simulink model "APCS"  (R2023a)
settings: Solver=VariableStepAuto  StartTime=0.0  StopTime=10.0  RelTol=1e-3
settings Model: Creator=asd19005  LastModifiedBy=aan18022

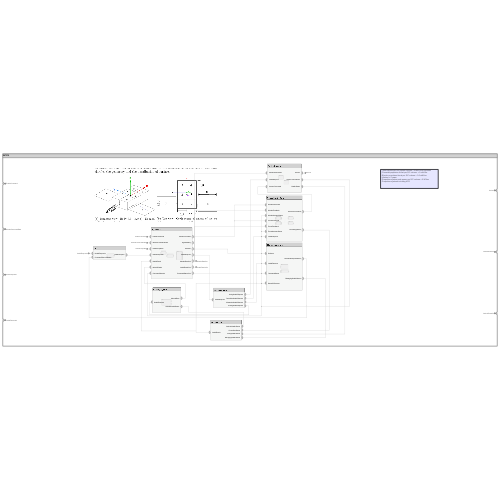
[thumbnail: Simulink's stored preview of the top-level diagram]
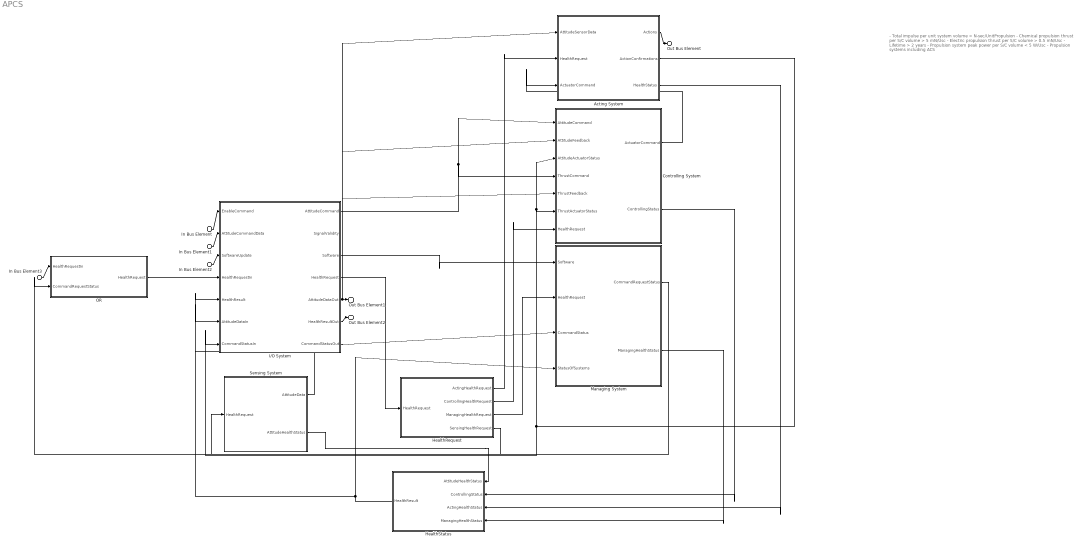
== system APCS ==
  note: - Total impulse per unit system volume > N-sec/UnitPropulsion
      | - Chemical propulsion thrust per S/C volume  > 5 mN/Usc
      | - Electric propulsion thrust per S/C volume > 0.5 mN/Usc
      | - Lifetime > 2 years
      | - Propulsion system peak power per S/C volume < 5 W/Usc
      | - Propulsion systems including ACS
  In Bus Element : Inport  PortName=EnableCommand
  In Bus Element1 : Inport  Port=2  PortName=AttitudeCommandData
  In Bus Element2 : Inport  Port=3  PortName=SoftwareUpdate
  In Bus Element3 : Inport  Port=4  PortName=HealthRequestIn
  Acting System : Subsystem
      settings: PortSchema="{\"entries\":[{\"content\":{\"headerSize\":26,\"margin\":15,\"minimumSpacing\":25,\"sides\":[{\"content\":{\"connectorIds\":[\"In1\",\"In2\",\"In3\"]},\"type\":\"ConnectorPlacement.EquallySpacedRectSide\",\"uuid\":\"fe9a0813-768f-43cf-a7a7-a35f6718a35e\"},{\"content\":{\"connectorIds\":[\"Out1\",\"Out2\",\"Out3\"],\"side\":\"RIGHT\"},\"type\":\"ConnectorPlacement.EquallySpacedRectSide\",\"uuid\":\"83a5fda2-f793-4516-8295-8e256804f86f\"},{\"content\":{\"side\":\"TOP\"},\"type\":\"ConnectorPlacement.EquallySpacedRectSide\",\"uuid\":\"9f7bc7bd-a98b-401f-acf1-cfd6a0f445f8\"}]},\"type\":\"ConnectorPlacement.EquallySpacedConnector\",\"uuid\":\"2641b729-a1f9-4d54-83a2-7f405081950a\"}],\"packageUris\":[\"http://schema.mathworks.com/mf0/Connector/R2020b\"],\"version\":\"1.0\"}"
  Controlling System : Subsystem
      settings: PortSchema="{\"entries\":[{\"content\":{\"headerSize\":26,\"margin\":15,\"minimumSpacing\":25,\"sides\":[{\"content\":{\"connectorIds\":[\"In1\",\"In5\",\"In3\",\"In2\",\"In6\",\"In4\",\"In7\"]},\"type\":\"ConnectorPlacement.EquallySpacedRectSide\",\"uuid\":\"fe9a0813-768f-43cf-a7a7-a35f6718a35e\"},{\"content\":{\"connectorIds\":[\"Out1\",\"Out2\"],\"side\":\"RIGHT\"},\"type\":\"ConnectorPlacement.EquallySpacedRectSide\",\"uuid\":\"83a5fda2-f793-4516-8295-8e256804f86f\"},{\"content\":{\"side\":\"TOP\"},\"type\":\"ConnectorPlacement.EquallySpacedRectSide\",\"uuid\":\"9f7bc7bd-a98b-401f-acf1-cfd6a0f445f8\"}]},\"type\":\"ConnectorPlacement.EquallySpacedConnector\",\"uuid\":\"2641b729-a1f9-4d54-83a2-7f405081950a\"}],\"packageUris\":[\"http://schema.mathworks.com/mf0/Connector/R2020b\"],\"version\":\"1.0\"}"
  HealthRequest : Subsystem
      settings: PortSchema="{\"entries\":[{\"content\":{\"headerSize\":26,\"margin\":15,\"minimumSpacing\":25,\"sides\":[{\"content\":{\"connectorIds\":[\"In1\"]},\"type\":\"ConnectorPlacement.EquallySpacedRectSide\",\"uuid\":\"fe9a0813-768f-43cf-a7a7-a35f6718a35e\"},{\"content\":{\"connectorIds\":[\"Out4\",\"Out1\",\"Out2\",\"Out3\"],\"side\":\"RIGHT\"},\"type\":\"ConnectorPlacement.EquallySpacedRectSide\",\"uuid\":\"83a5fda2-f793-4516-8295-8e256804f86f\"},{\"content\":{\"side\":\"TOP\"},\"type\":\"ConnectorPlacement.EquallySpacedRectSide\",\"uuid\":\"9f7bc7bd-a98b-401f-acf1-cfd6a0f445f8\"}]},\"type\":\"ConnectorPlacement.EquallySpacedConnector\",\"uuid\":\"2641b729-a1f9-4d54-83a2-7f405081950a\"}],\"packageUris\":[\"http://schema.mathworks.com/mf0/Connector/R2020b\"],\"version\":\"1.0\"}"
  HealthStatus : Subsystem
      settings: PortSchema="{\"entries\":[{\"content\":{\"headerSize\":26,\"margin\":15,\"minimumSpacing\":25,\"sides\":[{\"content\":{\"connectorIds\":[\"Out1\"]},\"type\":\"ConnectorPlacement.EquallySpacedRectSide\",\"uuid\":\"fe9a0813-768f-43cf-a7a7-a35f6718a35e\"},{\"content\":{\"connectorIds\":[\"In1\",\"In2\",\"In3\",\"In4\"],\"side\":\"RIGHT\"},\"type\":\"ConnectorPlacement.EquallySpacedRectSide\",\"uuid\":\"83a5fda2-f793-4516-8295-8e256804f86f\"},{\"content\":{\"side\":\"TOP\"},\"type\":\"ConnectorPlacement.EquallySpacedRectSide\",\"uuid\":\"9f7bc7bd-a98b-401f-acf1-cfd6a0f445f8\"}]},\"type\":\"ConnectorPlacement.EquallySpacedConnector\",\"uuid\":\"2641b729-a1f9-4d54-83a2-7f405081950a\"}],\"packageUris\":[\"http://schema.mathworks.com/mf0/Connector/R2020b\"],\"version\":\"1.0\"}"
  I/O System : Subsystem
      settings: PortSchema="{\"entries\":[{\"content\":{\"headerSize\":26,\"margin\":15,\"minimumSpacing\":25,\"sides\":[{\"content\":{\"connectorIds\":[\"In1\",\"In2\",\"In3\",\"In4\",\"In5\",\"In6\",\"In7\"]},\"type\":\"ConnectorPlacement.EquallySpacedRectSide\",\"uuid\":\"fe9a0813-768f-43cf-a7a7-a35f6718a35e\"},{\"content\":{\"connectorIds\":[\"Out1\",\"Out2\",\"Out3\",\"Out4\",\"Out5\",\"Out6\",\"Out7\"],\"side\":\"RIGHT\"},\"type\":\"ConnectorPlacement.EquallySpacedRectSide\",\"uuid\":\"83a5fda2-f793-4516-8295-8e256804f86f\"},{\"content\":{\"side\":\"TOP\"},\"type\":\"ConnectorPlacement.EquallySpacedRectSide\",\"uuid\":\"9f7bc7bd-a98b-401f-acf1-cfd6a0f445f8\"}]},\"type\":\"ConnectorPlacement.EquallySpacedConnector\",\"uuid\":\"2641b729-a1f9-4d54-83a2-7f405081950a\"}],\"packageUris\":[\"http://schema.mathworks.com/mf0/Connector/R2020b\"],\"version\":\"1.0\"}"
  Managing System : Subsystem
      settings: PortSchema="{\"entries\":[{\"content\":{\"headerSize\":26,\"margin\":15,\"minimumSpacing\":25,\"sides\":[{\"content\":{\"connectorIds\":[\"In1\",\"In2\",\"In3\",\"In4\"]},\"type\":\"ConnectorPlacement.EquallySpacedRectSide\",\"uuid\":\"fe9a0813-768f-43cf-a7a7-a35f6718a35e\"},{\"content\":{\"connectorIds\":[\"Out1\",\"Out2\"],\"side\":\"RIGHT\"},\"type\":\"ConnectorPlacement.EquallySpacedRectSide\",\"uuid\":\"83a5fda2-f793-4516-8295-8e256804f86f\"},{\"content\":{\"side\":\"TOP\"},\"type\":\"ConnectorPlacement.EquallySpacedRectSide\",\"uuid\":\"9f7bc7bd-a98b-401f-acf1-cfd6a0f445f8\"}]},\"type\":\"ConnectorPlacement.EquallySpacedConnector\",\"uuid\":\"2641b729-a1f9-4d54-83a2-7f405081950a\"}],\"packageUris\":[\"http://schema.mathworks.com/mf0/Connector/R2020b\"],\"version\":\"1.0\"}"
  OR : Subsystem
      settings: PortSchema="{\"entries\":[{\"content\":{\"headerSize\":26,\"margin\":15,\"minimumSpacing\":25,\"sides\":[{\"content\":{\"connectorIds\":[\"In2\",\"In1\"]},\"type\":\"ConnectorPlacement.EquallySpacedRectSide\",\"uuid\":\"fe9a0813-768f-43cf-a7a7-a35f6718a35e\"},{\"content\":{\"connectorIds\":[\"Out1\"],\"side\":\"RIGHT\"},\"type\":\"ConnectorPlacement.EquallySpacedRectSide\",\"uuid\":\"83a5fda2-f793-4516-8295-8e256804f86f\"},{\"content\":{\"side\":\"TOP\"},\"type\":\"ConnectorPlacement.EquallySpacedRectSide\",\"uuid\":\"9f7bc7bd-a98b-401f-acf1-cfd6a0f445f8\"}]},\"type\":\"ConnectorPlacement.EquallySpacedConnector\",\"uuid\":\"2641b729-a1f9-4d54-83a2-7f405081950a\"}],\"packageUris\":[\"http://schema.mathworks.com/mf0/Connector/R2020b\"],\"version\":\"1.0\"}"
  Sensing System : Subsystem
      settings: PortSchema="{\"entries\":[{\"content\":{\"headerSize\":26,\"margin\":15,\"minimumSpacing\":25,\"sides\":[{\"content\":{\"connectorIds\":[\"In1\"]},\"type\":\"ConnectorPlacement.EquallySpacedRectSide\",\"uuid\":\"fe9a0813-768f-43cf-a7a7-a35f6718a35e\"},{\"content\":{\"connectorIds\":[\"Out1\",\"Out2\"],\"side\":\"RIGHT\"},\"type\":\"ConnectorPlacement.EquallySpacedRectSide\",\"uuid\":\"83a5fda2-f793-4516-8295-8e256804f86f\"},{\"content\":{\"side\":\"TOP\"},\"type\":\"ConnectorPlacement.EquallySpacedRectSide\",\"uuid\":\"9f7bc7bd-a98b-401f-acf1-cfd6a0f445f8\"}]},\"type\":\"ConnectorPlacement.EquallySpacedConnector\",\"uuid\":\"2641b729-a1f9-4d54-83a2-7f405081950a\"}],\"packageUris\":[\"http://schema.mathworks.com/mf0/Connector/R2020b\"],\"version\":\"1.0\"}"
  Out Bus Element : Outport  PortName=Actions
  Out Bus Element2 : Outport  Port=2  PortName=HealthResultOut
  Out Bus Element1 : Outport  Port=3  PortName=AttitudeDataOut
  wires:
  In Bus Element/1 -> I/O System/1(EnableCommand)
  In Bus Element1/1 -> I/O System/2(AttitudeCommandData)
  In Bus Element2/1 -> I/O System/3(SoftwareUpdate)
  I/O System/1(AttitudeCommand) -> Controlling System/1(AttitudeCommand), Controlling System/2(ThrustCommand)
  I/O System/3(Software) -> Managing System/1(Software)
  Sensing System/1(AttitudeData) -> I/O System/6(AttitudeDataIn)
  Acting System/2(ActionConfirmations) -> Controlling System/3(AttitudeActuatorStatus), Controlling System/4(ThrustActuatorStatus), I/O System/7(CommandStatusIn)
  I/O System/5(AttitudeDataOut) -> Controlling System/5(AttitudeFeedback), Acting System/1(AttitudeSensorData), Controlling System/6(ThrustFeedback), Out Bus Element1/1
  I/O System/7(CommandStatusOut) -> Managing System/3(CommandStatus)
  Controlling System/1(ActuatorCommand) -> Acting System/3(ActuatorCommand)
  Acting System/1(Actions) -> Out Bus Element/1
  I/O System/6(HealthResultOut) -> Out Bus Element2/1
  I/O System/4(HealthRequest) -> HealthRequest/1(HealthRequest)
  HealthRequest/1(ControllingHealthRequest) -> Controlling System/7(HealthRequest)
  HealthRequest/2(ManagingHealthRequest) -> Managing System/2(HealthRequest)
  HealthRequest/4(ActingHealthRequest) -> Acting System/2(HealthRequest)
  HealthStatus/1(HealthResult) -> Managing System/4(StatusOfSystems), I/O System/5(HealthResult)
  HealthRequest/3(SensingHealthRequest) -> Sensing System/1(HealthRequest)
  Acting System/3(HealthStatus) -> HealthStatus/3(ActingHealthStatus)
  Managing System/2(ManagingHealthStatus) -> HealthStatus/4(ManagingHealthStatus)
  Controlling System/2(ControllingStatus) -> HealthStatus/2(ControllingStatus)
  In Bus Element3/1 -> OR/2(HealthRequestIn)
  Managing System/1(CommandRequestStatus) -> OR/1(CommandRequestStatus)
  OR/1(HealthRequest) -> I/O System/4(HealthRequestIn)
  Sensing System/2(AttitudeHealthStatus) -> HealthStatus/1(AttitudeHealthStatus)

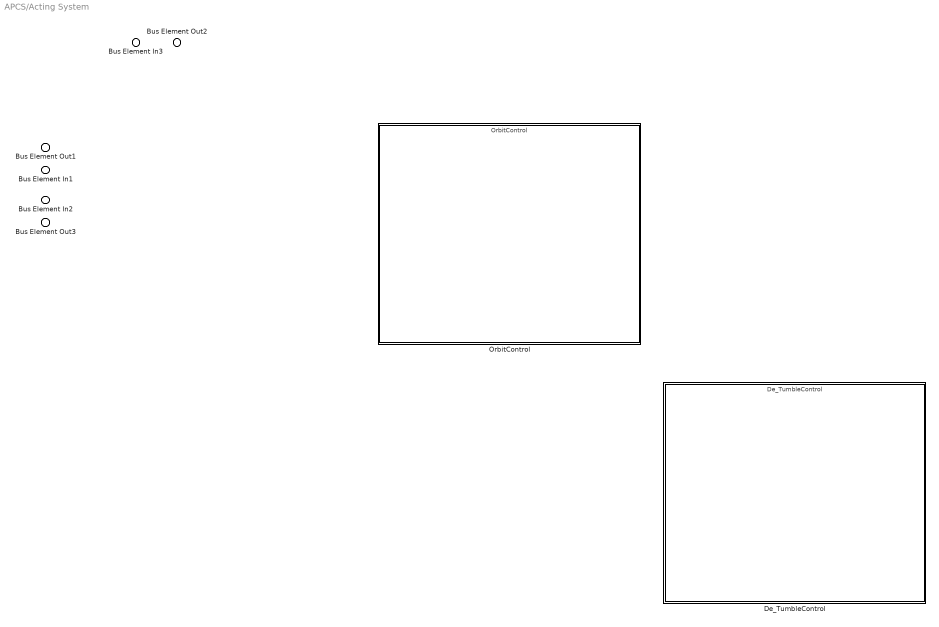
== system APCS/Acting System ==
  Bus Element In1 : Inport  PortName=AttitudeSensorData
  Bus Element In3 : Inport  Port=2  PortName=HealthRequest
  Bus Element In2 : Inport  Port=3  PortName=ActuatorCommand
  De_TumbleControl : ModelReference  ModelNameDialog=De_TumbleControl  SimulationMode=Normal  ModelReferenceVersion=1.0
      settings: PortSchema="{\"entries\":[{\"content\":{\"headerSize\":38,\"margin\":15,\"minimumSpacing\":25,\"sides\":[{\"content\":{},\"type\":\"ConnectorPlacement.EquallySpacedRectSide\",\"uuid\":\"e3457a29-b43c-4933-8a11-68e017a647c4\"},{\"content\":{\"side\":\"RIGHT\"},\"type\":\"ConnectorPlacement.EquallySpacedRectSide\",\"uuid\":\"7dfa2731-a543-4e50-aed6-e868771da571\"},{\"content\":{\"side\":\"TOP\"},\"type\":\"ConnectorPlacement.EquallySpacedRectSide\",\"uuid\":\"66e179e8-d7ed-4bc5-a0bd-f79bc464d9fe\"}]},\"type\":\"ConnectorPlacement.EquallySpacedConnector\",\"uuid\":\"61bb093a-de12-4127-8c6a-9ae2c62bada7\"}],\"packageUris\":[\"http://schema.mathworks.com/mf0/Connector/R2020b\"],\"version\":\"1.0\"}"
  OrbitControl : ModelReference  ModelNameDialog=OrbitControl  SimulationMode=Normal  ModelReferenceVersion=1.0
      settings: PortSchema="{\"entries\":[{\"content\":{\"headerSize\":38,\"margin\":15,\"minimumSpacing\":25,\"sides\":[{\"content\":{},\"type\":\"ConnectorPlacement.EquallySpacedRectSide\",\"uuid\":\"e3457a29-b43c-4933-8a11-68e017a647c4\"},{\"content\":{\"side\":\"RIGHT\"},\"type\":\"ConnectorPlacement.EquallySpacedRectSide\",\"uuid\":\"7dfa2731-a543-4e50-aed6-e868771da571\"},{\"content\":{\"side\":\"TOP\"},\"type\":\"ConnectorPlacement.EquallySpacedRectSide\",\"uuid\":\"66e179e8-d7ed-4bc5-a0bd-f79bc464d9fe\"}]},\"type\":\"ConnectorPlacement.EquallySpacedConnector\",\"uuid\":\"61bb093a-de12-4127-8c6a-9ae2c62bada7\"}],\"packageUris\":[\"http://schema.mathworks.com/mf0/Connector/R2020b\"],\"version\":\"1.0\"}"
  Bus Element Out2 : Outport  PortName=Actions
  Bus Element Out1 : Outport  Port=2  PortName=ActionConfirmations
  Bus Element Out3 : Outport  Port=3  PortName=HealthStatus

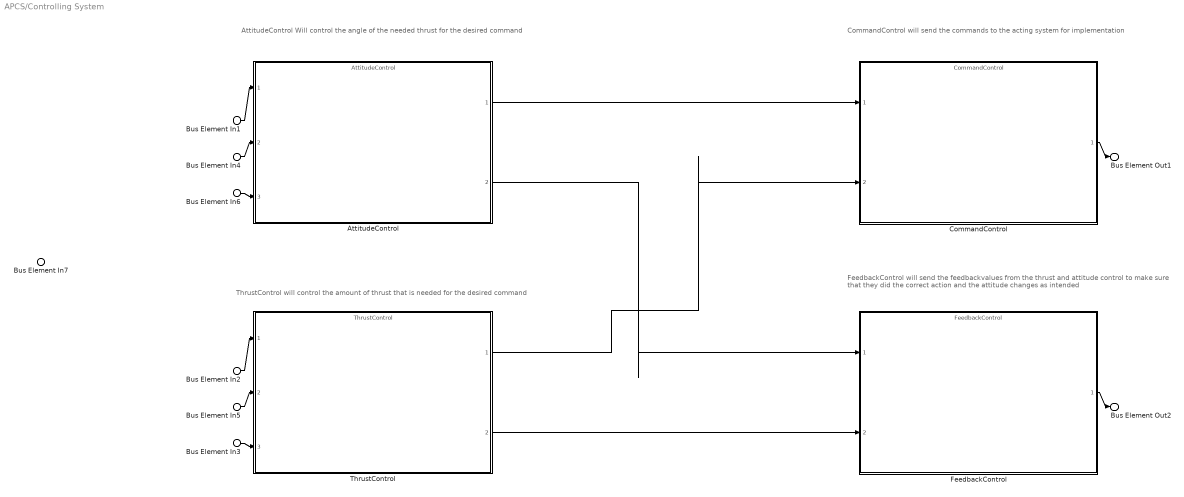
== system APCS/Controlling System ==
  note: CommandControl will send the commands to the acting system for implementation
  note: ThrustControl will control the amount of thrust that is needed for the desired command
  note: AttitudeControl Will control the angle of the needed thrust for the desired command
  note: FeedbackControl will send the feedbackvalues from the thrust and attitude control to make sure that they did the correct action and the attitude changes as intended
  Bus Element In1 : Inport  PortName=AttitudeCommand
  Bus Element In2 : Inport  Port=2  PortName=ThrustCommand
  Bus Element In6 : Inport  Port=3  PortName=AttitudeActuatorStatus
  Bus Element In3 : Inport  Port=4  PortName=ThrustActuatorStatus
  Bus Element In4 : Inport  Port=5  PortName=AttitudeFeedback
  Bus Element In5 : Inport  Port=6  PortName=ThrustFeedback
  Bus Element In7 : Inport  Port=7  PortName=HealthRequest
  AttitudeControl : ModelReference  ModelNameDialog=AttitudeControl.slx  SimulationMode=Normal  ModelReferenceVersion=1.1
      settings: PortSchema="{\"entries\":[{\"content\":{\"headerSize\":38,\"margin\":15,\"minimumSpacing\":25,\"sides\":[{\"content\":{\"connectorIds\":[\"In1\",\"In2\",\"In3\"]},\"type\":\"ConnectorPlacement.EquallySpacedRectSide\",\"uuid\":\"e3457a29-b43c-4933-8a11-68e017a647c4\"},{\"content\":{\"connectorIds\":[\"Out1\",\"Out2\"],\"side\":\"RIGHT\"},\"type\":\"ConnectorPlacement.EquallySpacedRectSide\",\"uuid\":\"7dfa2731-a543-4e50-aed6-e868771da571\"},{\"content\":{\"side\":\"TOP\"},\"type\":\"ConnectorPlacement.EquallySpacedRectSide\",\"uuid\":\"66e179e8-d7ed-4bc5-a0bd-f79bc464d9fe\"}]},\"type\":\"ConnectorPlacement.EquallySpacedConnector\",\"uuid\":\"61bb093a-de12-4127-8c6a-9ae2c62bada7\"}],\"packageUris\":[\"http://schema.mathworks.com/mf0/Connector/R2020b\"],\"version\":\"1.0\"}"
  CommandControl : ModelReference  ModelNameDialog=CommandControl  SimulationMode=Normal  ModelReferenceVersion=1.1
      settings: PortSchema="{\"entries\":[{\"content\":{\"headerSize\":38,\"margin\":15,\"minimumSpacing\":25,\"sides\":[{\"content\":{\"connectorIds\":[\"In1\",\"In2\"]},\"type\":\"ConnectorPlacement.EquallySpacedRectSide\",\"uuid\":\"e3457a29-b43c-4933-8a11-68e017a647c4\"},{\"content\":{\"connectorIds\":[\"Out1\"],\"side\":\"RIGHT\"},\"type\":\"ConnectorPlacement.EquallySpacedRectSide\",\"uuid\":\"7dfa2731-a543-4e50-aed6-e868771da571\"},{\"content\":{\"side\":\"TOP\"},\"type\":\"ConnectorPlacement.EquallySpacedRectSide\",\"uuid\":\"66e179e8-d7ed-4bc5-a0bd-f79bc464d9fe\"}]},\"type\":\"ConnectorPlacement.EquallySpacedConnector\",\"uuid\":\"61bb093a-de12-4127-8c6a-9ae2c62bada7\"}],\"packageUris\":[\"http://schema.mathworks.com/mf0/Connector/R2020b\"],\"version\":\"1.0\"}"
  FeedbackControl : ModelReference  ModelNameDialog=FeedbackControl  SimulationMode=Normal  ModelReferenceVersion=1.1
      settings: PortSchema="{\"entries\":[{\"content\":{\"headerSize\":38,\"margin\":15,\"minimumSpacing\":25,\"sides\":[{\"content\":{\"connectorIds\":[\"In1\",\"In2\"]},\"type\":\"ConnectorPlacement.EquallySpacedRectSide\",\"uuid\":\"e3457a29-b43c-4933-8a11-68e017a647c4\"},{\"content\":{\"connectorIds\":[\"Out1\"],\"side\":\"RIGHT\"},\"type\":\"ConnectorPlacement.EquallySpacedRectSide\",\"uuid\":\"7dfa2731-a543-4e50-aed6-e868771da571\"},{\"content\":{\"side\":\"TOP\"},\"type\":\"ConnectorPlacement.EquallySpacedRectSide\",\"uuid\":\"66e179e8-d7ed-4bc5-a0bd-f79bc464d9fe\"}]},\"type\":\"ConnectorPlacement.EquallySpacedConnector\",\"uuid\":\"61bb093a-de12-4127-8c6a-9ae2c62bada7\"}],\"packageUris\":[\"http://schema.mathworks.com/mf0/Connector/R2020b\"],\"version\":\"1.0\"}"
  ThrustControl : ModelReference  ModelNameDialog=ThrustControl  SimulationMode=Normal  ModelReferenceVersion=1.1
      settings: PortSchema="{\"entries\":[{\"content\":{\"headerSize\":38,\"margin\":15,\"minimumSpacing\":25,\"sides\":[{\"content\":{\"connectorIds\":[\"In1\",\"In2\",\"In3\"]},\"type\":\"ConnectorPlacement.EquallySpacedRectSide\",\"uuid\":\"e3457a29-b43c-4933-8a11-68e017a647c4\"},{\"content\":{\"connectorIds\":[\"Out1\",\"Out2\"],\"side\":\"RIGHT\"},\"type\":\"ConnectorPlacement.EquallySpacedRectSide\",\"uuid\":\"7dfa2731-a543-4e50-aed6-e868771da571\"},{\"content\":{\"side\":\"TOP\"},\"type\":\"ConnectorPlacement.EquallySpacedRectSide\",\"uuid\":\"66e179e8-d7ed-4bc5-a0bd-f79bc464d9fe\"}]},\"type\":\"ConnectorPlacement.EquallySpacedConnector\",\"uuid\":\"61bb093a-de12-4127-8c6a-9ae2c62bada7\"}],\"packageUris\":[\"http://schema.mathworks.com/mf0/Connector/R2020b\"],\"version\":\"1.0\"}"
  Bus Element Out1 : Outport  PortName=ActuatorCommand
  Bus Element Out2 : Outport  Port=2  PortName=ControllingStatus
  wires:
  Bus Element In6/1 -> AttitudeControl/3
  Bus Element In1/1 -> AttitudeControl/1
  Bus Element In4/1 -> AttitudeControl/2
  Bus Element In3/1 -> ThrustControl/3
  Bus Element In2/1 -> ThrustControl/1
  Bus Element In5/1 -> ThrustControl/2
  AttitudeControl/1 -> CommandControl/1
  ThrustControl/1 -> CommandControl/2
  CommandControl/1 -> Bus Element Out1/1
  AttitudeControl/2 -> FeedbackControl/1
  ThrustControl/2 -> FeedbackControl/2
  FeedbackControl/1 -> Bus Element Out2/1

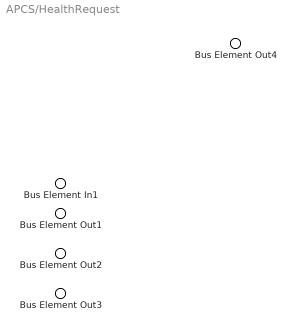
== system APCS/HealthRequest ==
  Bus Element In1 : Inport  PortName=HealthRequest
  Bus Element Out1 : Outport  PortName=ControllingHealthRequest
  Bus Element Out2 : Outport  Port=2  PortName=ManagingHealthRequest
  Bus Element Out4 : Outport  Port=3  PortName=SensingHealthRequest
  Bus Element Out3 : Outport  Port=4  PortName=ActingHealthRequest

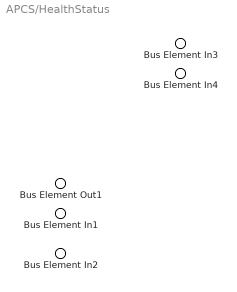
== system APCS/HealthStatus ==
  Bus Element In4 : Inport  PortName=AttitudeHealthStatus
  Bus Element In3 : Inport  Port=2  PortName=ControllingStatus
  Bus Element In1 : Inport  Port=3  PortName=ActingHealthStatus
  Bus Element In2 : Inport  Port=4  PortName=ManagingHealthStatus
  Bus Element Out1 : Outport  PortName=HealthResult

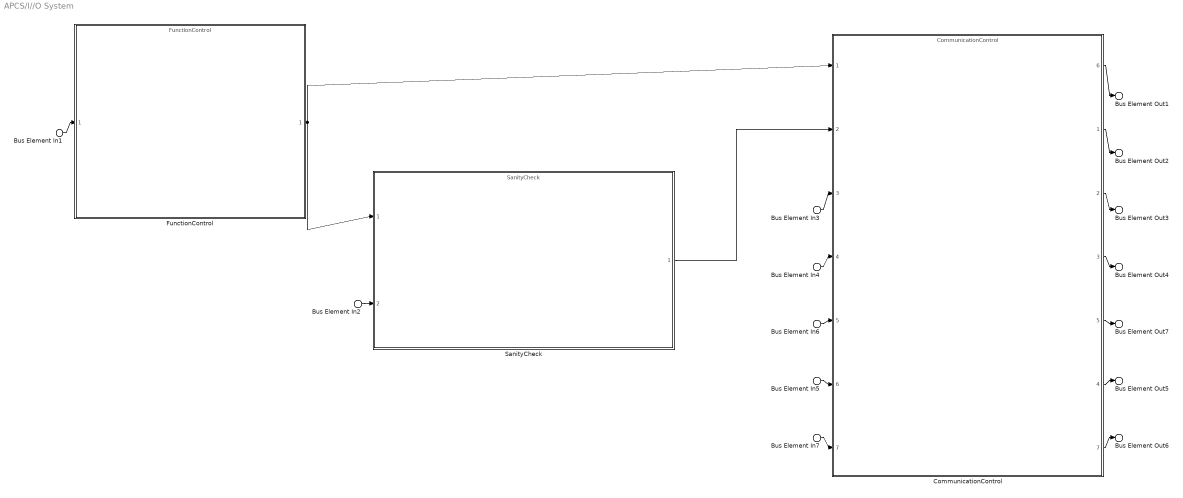
== system APCS/I//O System ==
  Bus Element In1 : Inport  PortName=EnableCommand
  Bus Element In2 : Inport  Port=2  PortName=AttitudeCommandData
  Bus Element In3 : Inport  Port=3  PortName=SoftwareUpdate
  Bus Element In4 : Inport  Port=4  PortName=HealthRequestIn
  Bus Element In6 : Inport  Port=5  PortName=HealthResult
  Bus Element In5 : Inport  Port=6  PortName=AttitudeDataIn
  Bus Element In7 : Inport  Port=7  PortName=CommandStatusIn
  CommunicationControl : ModelReference  ModelNameDialog=CommunicationControl  SimulationMode=Normal  ModelReferenceVersion=1.2
      settings: PortSchema="{\"entries\":[{\"content\":{\"headerSize\":38,\"margin\":15,\"minimumSpacing\":25,\"sides\":[{\"content\":{\"connectorIds\":[\"In1\",\"In2\",\"In3\",\"In4\",\"In5\",\"In6\",\"In7\"]},\"type\":\"ConnectorPlacement.EquallySpacedRectSide\",\"uuid\":\"e3457a29-b43c-4933-8a11-68e017a647c4\"},{\"content\":{\"connectorIds\":[\"Out6\",\"Out1\",\"Out2\",\"Out3\",\"Out5\",\"Out4\",\"Out7\"],\"side\":\"RIGHT\"},\"type\":\"ConnectorPlacement.EquallySpacedRectSide\",\"uuid\":\"7dfa2731-a543-4e50-aed6-e868771da571\"},{\"content\":{\"side\":\"TOP\"},\"type\":\"ConnectorPlacement.EquallySpacedRectSide\",\"uuid\":\"66e179e8-d7ed-4bc5-a0bd-f79bc464d9fe\"}]},\"type\":\"ConnectorPlacement.EquallySpacedConnector\",\"uuid\":\"61bb093a-de12-4127-8c6a-9ae2c62bada7\"}],\"packageUris\":[\"http://schema.mathworks.com/mf0/Connector/R2020b\"],\"version\":\"1.0\"}"
  FunctionControl : ModelReference  ModelNameDialog=FunctionControl  SimulationMode=Normal  ModelReferenceVersion=1.2
      settings: PortSchema="{\"entries\":[{\"content\":{\"headerSize\":38,\"margin\":15,\"minimumSpacing\":25,\"sides\":[{\"content\":{\"connectorIds\":[\"In1\"]},\"type\":\"ConnectorPlacement.EquallySpacedRectSide\",\"uuid\":\"e3457a29-b43c-4933-8a11-68e017a647c4\"},{\"content\":{\"connectorIds\":[\"Out1\"],\"side\":\"RIGHT\"},\"type\":\"ConnectorPlacement.EquallySpacedRectSide\",\"uuid\":\"7dfa2731-a543-4e50-aed6-e868771da571\"},{\"content\":{\"side\":\"TOP\"},\"type\":\"ConnectorPlacement.EquallySpacedRectSide\",\"uuid\":\"66e179e8-d7ed-4bc5-a0bd-f79bc464d9fe\"}]},\"type\":\"ConnectorPlacement.EquallySpacedConnector\",\"uuid\":\"61bb093a-de12-4127-8c6a-9ae2c62bada7\"}],\"packageUris\":[\"http://schema.mathworks.com/mf0/Connector/R2020b\"],\"version\":\"1.0\"}"
  SanityCheck : ModelReference  ModelNameDialog=SanityCheck  SimulationMode=Normal  ModelReferenceVersion=1.2
      settings: PortSchema="{\"entries\":[{\"content\":{\"headerSize\":38,\"margin\":15,\"minimumSpacing\":25,\"sides\":[{\"content\":{\"connectorIds\":[\"In1\",\"In2\"]},\"type\":\"ConnectorPlacement.EquallySpacedRectSide\",\"uuid\":\"e3457a29-b43c-4933-8a11-68e017a647c4\"},{\"content\":{\"connectorIds\":[\"Out1\"],\"side\":\"RIGHT\"},\"type\":\"ConnectorPlacement.EquallySpacedRectSide\",\"uuid\":\"7dfa2731-a543-4e50-aed6-e868771da571\"},{\"content\":{\"side\":\"TOP\"},\"type\":\"ConnectorPlacement.EquallySpacedRectSide\",\"uuid\":\"66e179e8-d7ed-4bc5-a0bd-f79bc464d9fe\"}]},\"type\":\"ConnectorPlacement.EquallySpacedConnector\",\"uuid\":\"61bb093a-de12-4127-8c6a-9ae2c62bada7\"}],\"packageUris\":[\"http://schema.mathworks.com/mf0/Connector/R2020b\"],\"version\":\"1.0\"}"
  Bus Element Out1 : Outport  PortName=AttitudeCommand
  Bus Element Out2 : Outport  Port=2  PortName=SignalValidity
  Bus Element Out3 : Outport  Port=3  PortName=Software
  Bus Element Out4 : Outport  Port=4  PortName=HealthRequest
  Bus Element Out5 : Outport  Port=5  PortName=AttitudeDataOut
  Bus Element Out7 : Outport  Port=6  PortName=HealthResultOut
  Bus Element Out6 : Outport  Port=7  PortName=CommandStatusOut
  wires:
  Bus Element In1/1 -> FunctionControl/1
  FunctionControl/1 -> SanityCheck/1, CommunicationControl/1
  Bus Element In2/1 -> SanityCheck/2
  SanityCheck/1 -> CommunicationControl/2
  Bus Element In5/1 -> CommunicationControl/6
  Bus Element In7/1 -> CommunicationControl/7
  Bus Element In4/1 -> CommunicationControl/4
  Bus Element In6/1 -> CommunicationControl/5
  Bus Element In3/1 -> CommunicationControl/3
  CommunicationControl/6 -> Bus Element Out1/1
  CommunicationControl/4 -> Bus Element Out5/1
  CommunicationControl/7 -> Bus Element Out6/1
  CommunicationControl/3 -> Bus Element Out4/1
  CommunicationControl/5 -> Bus Element Out7/1
  CommunicationControl/1 -> Bus Element Out2/1
  CommunicationControl/2 -> Bus Element Out3/1

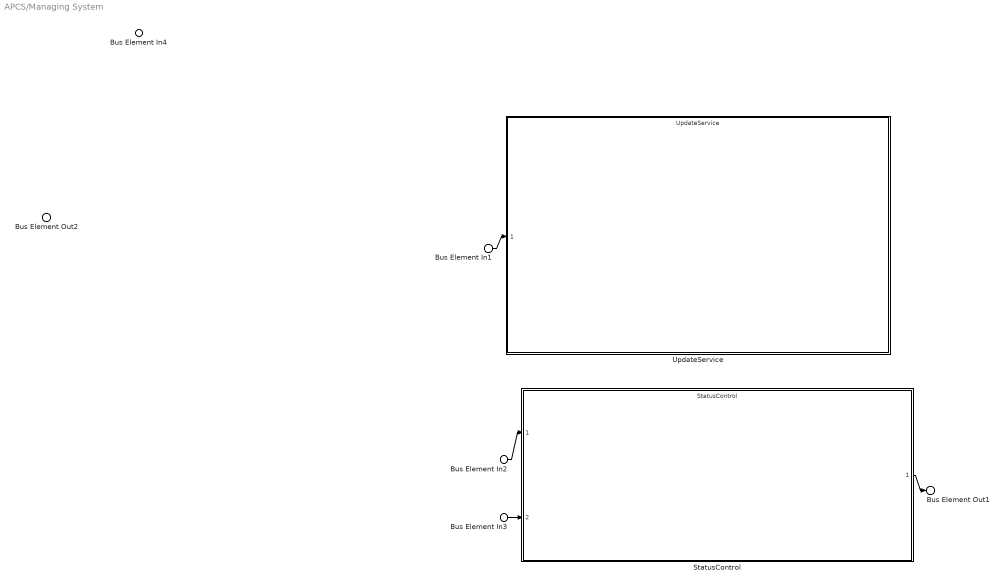
== system APCS/Managing System ==
  Bus Element In1 : Inport  PortName=Software
  Bus Element In4 : Inport  Port=2  PortName=HealthRequest
  Bus Element In2 : Inport  Port=3  PortName=CommandStatus
  Bus Element In3 : Inport  Port=4  PortName=StatusOfSystems
  StatusControl : ModelReference  ModelNameDialog=StatusControl  SimulationMode=Normal  ModelReferenceVersion=1.1
      settings: PortSchema="{\"entries\":[{\"content\":{\"headerSize\":38,\"margin\":15,\"minimumSpacing\":25,\"sides\":[{\"content\":{\"connectorIds\":[\"In1\",\"In2\"]},\"type\":\"ConnectorPlacement.EquallySpacedRectSide\",\"uuid\":\"e3457a29-b43c-4933-8a11-68e017a647c4\"},{\"content\":{\"connectorIds\":[\"Out1\"],\"side\":\"RIGHT\"},\"type\":\"ConnectorPlacement.EquallySpacedRectSide\",\"uuid\":\"7dfa2731-a543-4e50-aed6-e868771da571\"},{\"content\":{\"side\":\"TOP\"},\"type\":\"ConnectorPlacement.EquallySpacedRectSide\",\"uuid\":\"66e179e8-d7ed-4bc5-a0bd-f79bc464d9fe\"}]},\"type\":\"ConnectorPlacement.EquallySpacedConnector\",\"uuid\":\"61bb093a-de12-4127-8c6a-9ae2c62bada7\"}],\"packageUris\":[\"http://schema.mathworks.com/mf0/Connector/R2020b\"],\"version\":\"1.0\"}"
  UpdateService : ModelReference  ModelNameDialog=UpdateService  SimulationMode=Normal  ModelReferenceVersion=1.1
      settings: PortSchema="{\"entries\":[{\"content\":{\"headerSize\":38,\"margin\":15,\"minimumSpacing\":25,\"sides\":[{\"content\":{\"connectorIds\":[\"In1\"]},\"type\":\"ConnectorPlacement.EquallySpacedRectSide\",\"uuid\":\"e3457a29-b43c-4933-8a11-68e017a647c4\"},{\"content\":{\"side\":\"RIGHT\"},\"type\":\"ConnectorPlacement.EquallySpacedRectSide\",\"uuid\":\"7dfa2731-a543-4e50-aed6-e868771da571\"},{\"content\":{\"side\":\"TOP\"},\"type\":\"ConnectorPlacement.EquallySpacedRectSide\",\"uuid\":\"66e179e8-d7ed-4bc5-a0bd-f79bc464d9fe\"}]},\"type\":\"ConnectorPlacement.EquallySpacedConnector\",\"uuid\":\"61bb093a-de12-4127-8c6a-9ae2c62bada7\"}],\"packageUris\":[\"http://schema.mathworks.com/mf0/Connector/R2020b\"],\"version\":\"1.0\"}"
  Bus Element Out1 : Outport  PortName=CommandRequestStatus
  Bus Element Out2 : Outport  Port=2  PortName=ManagingHealthStatus
  wires:
  Bus Element In1/1 -> UpdateService/1
  Bus Element In2/1 -> StatusControl/1
  Bus Element In3/1 -> StatusControl/2
  StatusControl/1 -> Bus Element Out1/1

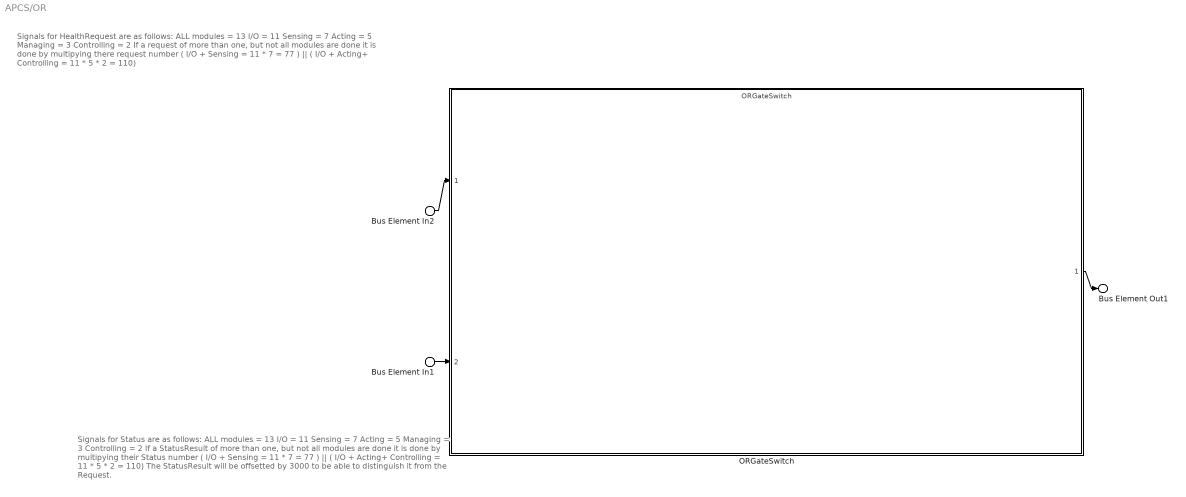
== system APCS/OR ==
  note: Signals for HealthRequest are as follows: ALL modules	= 13
      | 												I/O 	= 11
      | 											Sensing 	= 7
      | 											Acting	= 5
      | 										Managing	= 3
      | 										Controlling	= 2
      | If a request of more than one, but not all modules are done it is done by multipying there request number
      | ( I/O + Sensing = 11 * 7 = 77 ) || ( I/O + Acting+ Controlling = 11 * 5 * 2 = 110)
  note: Signals for Status are as follows:                    ALL modules = 13
      | 											        I/O	= 11
      | 											Sensing 	= 7
      | 											   Acting 	= 5
      | 										    Managing	= 3
      | 										   Controlling	= 2
      | If a StatusResult of more than one, but not all modules are done it is done by multipying their Status number
      | ( I/O + Sensing = 11 * 7 = 77 ) || ( I/O + Acting+ Controlling = 11 * 5 * 2 = 110)
      | The StatusResult will be offsetted by 3000 to be able to distinguish it from the Request.
  Bus Element In1 : Inport  PortName=CommandRequestStatus
  Bus Element In2 : Inport  Port=2  PortName=HealthRequestIn
  ORGateSwitch : ModelReference  ModelNameDialog=ORGateSwitch.slx  SimulationMode=Normal  ModelReferenceVersion=1.6
      settings: PortSchema="{\"entries\":[{\"content\":{\"headerSize\":38,\"margin\":15,\"minimumSpacing\":25,\"sides\":[{\"content\":{\"connectorIds\":[\"In1\",\"In2\"]},\"type\":\"ConnectorPlacement.EquallySpacedRectSide\",\"uuid\":\"e3457a29-b43c-4933-8a11-68e017a647c4\"},{\"content\":{\"connectorIds\":[\"Out1\"],\"side\":\"RIGHT\"},\"type\":\"ConnectorPlacement.EquallySpacedRectSide\",\"uuid\":\"7dfa2731-a543-4e50-aed6-e868771da571\"},{\"content\":{\"side\":\"TOP\"},\"type\":\"ConnectorPlacement.EquallySpacedRectSide\",\"uuid\":\"66e179e8-d7ed-4bc5-a0bd-f79bc464d9fe\"}]},\"type\":\"ConnectorPlacement.EquallySpacedConnector\",\"uuid\":\"61bb093a-de12-4127-8c6a-9ae2c62bada7\"}],\"packageUris\":[\"http://schema.mathworks.com/mf0/Connector/R2020b\"],\"version\":\"1.0\"}"
  Bus Element Out1 : Outport  PortName=HealthRequest
  wires:
  Bus Element In1/1 -> ORGateSwitch/2
  Bus Element In2/1 -> ORGateSwitch/1
  ORGateSwitch/1 -> Bus Element Out1/1

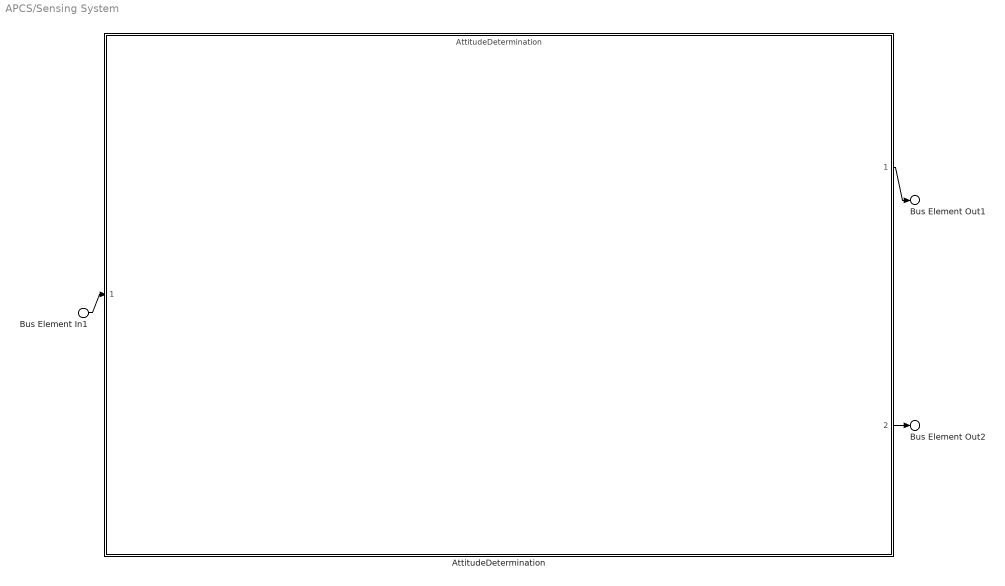
== system APCS/Sensing System ==
  Bus Element In1 : Inport  PortName=HealthRequest
  AttitudeDetermination : ModelReference  ModelNameDialog=AttitudeDetermination  SimulationMode=Normal  ModelReferenceVersion=1.2
      settings: PortSchema="{\"entries\":[{\"content\":{\"headerSize\":38,\"margin\":15,\"minimumSpacing\":25,\"sides\":[{\"content\":{\"connectorIds\":[\"In1\"]},\"type\":\"ConnectorPlacement.EquallySpacedRectSide\",\"uuid\":\"e3457a29-b43c-4933-8a11-68e017a647c4\"},{\"content\":{\"connectorIds\":[\"Out1\",\"Out2\"],\"side\":\"RIGHT\"},\"type\":\"ConnectorPlacement.EquallySpacedRectSide\",\"uuid\":\"7dfa2731-a543-4e50-aed6-e868771da571\"},{\"content\":{\"side\":\"TOP\"},\"type\":\"ConnectorPlacement.EquallySpacedRectSide\",\"uuid\":\"66e179e8-d7ed-4bc5-a0bd-f79bc464d9fe\"}]},\"type\":\"ConnectorPlacement.EquallySpacedConnector\",\"uuid\":\"61bb093a-de12-4127-8c6a-9ae2c62bada7\"}],\"packageUris\":[\"http://schema.mathworks.com/mf0/Connector/R2020b\"],\"version\":\"1.0\"}"
  Bus Element Out1 : Outport  PortName=AttitudeData
  Bus Element Out2 : Outport  Port=2  PortName=AttitudeHealthStatus
  wires:
  Bus Element In1/1 -> AttitudeDetermination/1
  AttitudeDetermination/1 -> Bus Element Out1/1
  AttitudeDetermination/2 -> Bus Element Out2/1
